simulink model "svpwm_inv_Motor_new_sent_split4_myMod1_simplified_free"  (R2023a)
settings: Solver=daessc  StartTime=0.0  StopTime=1  MaxStep=2.5e-7  RelTol=1e-3
libraries: fl_lib x17, nesl_utility x11, ee_lib x1, simulink x1
settings Model: SimulationMode=rapid-accelerator  Creator=alexey  LastModifiedBy=alexey
settings SolverCC: ZeroCrossAlgorithm=Adaptive
settings OptimizationCC: ReuseModelBlockBuffer=off
settings DebuggingCC: IgnoredZcDiagnostic=none
settings GRTTargetCC: RTWCAPISignals=on  RTWCAPIParams=on

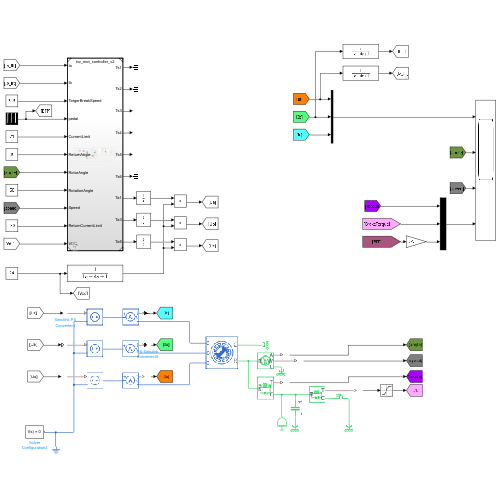
[thumbnail: Simulink's stored preview of the top-level diagram]
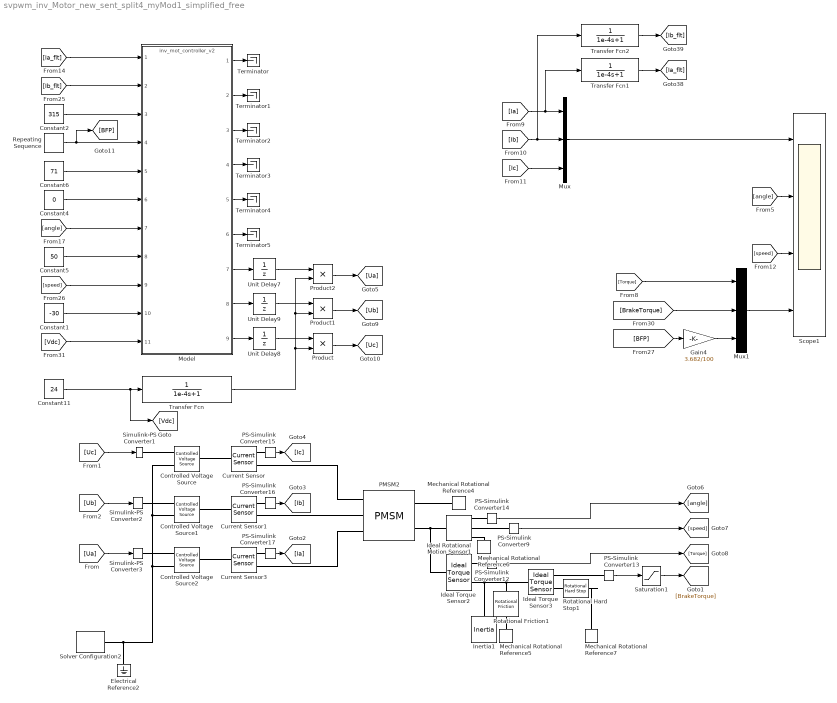
== system svpwm_inv_Motor_new_sent_split4_myMod1_simplified_free ==
  Constant1 : Constant  Value=-30
  Constant11 : Constant  Value=24
  Constant2 : Constant  Value=315
  Constant4 : Constant  Value=0
  Constant5 : Constant  Value=50
  Constant6 : Constant  Value=71
  Controlled Voltage Source : fl_lib/Electrical/Electrical Sources/Controlled Voltage Source
  Controlled Voltage Source1 : fl_lib/Electrical/Electrical Sources/Controlled Voltage Source
  Controlled Voltage Source2 : fl_lib/Electrical/Electrical Sources/Controlled Voltage Source
  Current Sensor : fl_lib/Electrical/Electrical Sensors/Current Sensor
  Current Sensor1 : fl_lib/Electrical/Electrical Sensors/Current Sensor
  Current Sensor3 : fl_lib/Electrical/Electrical Sensors/Current Sensor
  Electrical Reference2 : fl_lib/Electrical/Electrical Elements/Electrical Reference
  Gain4 : Gain  Gain=3.682/100
  Ideal Rotational Motion Sensor1 : fl_lib/Mechanical/Mechanical Sensors/Ideal Rotational Motion Sensor  reference=foundation.enum.MeasurementReference.difference  acceleration_port=false  velocity_port=true  position_port=true  wrap_angle=false  offset=0 rad
  Ideal Torque Sensor2 : fl_lib/Mechanical/Mechanical Sensors/Ideal Torque Sensor
  Ideal Torque Sensor3 : fl_lib/Mechanical/Mechanical Sensors/Ideal Torque Sensor
  Inertia1 : fl_lib/Mechanical/Rotational Elements/Inertia  inertia=3e-5 kg*m^2  num_ports=foundation.enum.numPorts2.one  w_specify=on  w_priority=High  w=0 rad/s  w_nominal_specify=off  w_nominal_unit=rad/s  w_nominal_value=1  t_specify=off  t_priority=None  t=0 N*m  t_nominal_specify=off  t_nominal_unit=N*m  t_nominal_value=1
  Mechanical Rotational Reference{4..7} (4 alike) : fl_lib/Mechanical/Rotational Elements/Mechanical Rotational Reference
  Model : ModelReference  ModelNameDialog=inv_mot_controller_v2.slx  SimulationMode=Normal  ModelReferenceVersion=1.6
  Mux : Mux  Inputs=3
  Mux1 : Mux  Inputs=3
  PMSM2 : ee_lib/Electromechanical/Permanent Magnet/PMSM  port_option=ee.enum.threePhasePort.expanded  winding_type=ee.enum.statorconnection.delta  machine_param=ee.enum.pmsm.parameterization.constant  nPolePairs=4  pmflux_param=ee.enum.pmflux.fluxlinkage  pm_flux_linkage=0.0163 Wb  torque_constant=0.074 N*m/A  back_emf_constant=0.06 V*s/rad  stator_param=ee.enum.statorparam.LdLqL0  Ld=119 uH  Lq=167 uH  idVec=[-200, 0, 200] A  iqVec=[-200, 0, 200] A  LdMatrix=0.0002 * ones(3, 3) H  LqMatrix=0.0002 * ones(3, 3) H  PmMatrix=0.1 * ones(3, 3) Wb  ktMatrix=0.18 * ones(3, 3) N*m/A  keMatrix=0.18 * ones(3, 3) V*s/rad  L0=1e-6 uH  Ls=0.0002 H  Lm=-0.00002 H  Ms=0.00002 H  Rs=0.1 Ohm  zero_sequence=ee.enum.park.zerosequence.include  axes_param=ee.enum.rotorangle.daxis  loss_param=ee.enum.ironloss.none  losses_oc=[0, 0, 0] W  losses_sc=[0, 0, 0] W  f_losses=60 Hz  Isc_losses=95 A  J=1e-8 kg*m^2  lam=0.00005 N*m*s/rad  i_d_specify=on  i_d_priority=None  i_d=0 A  i_d_nominal_specify=off  i_d_nominal_unit=A  i_d_nominal_value=1  i_q_specify=on  i_q_priority=None  i_q=0 A  i_q_nominal_specify=off  i_q_nominal_unit=A  i_q_nominal_value=1  torque_specify=on  torque_priority=None  torque=0 N*m  torque_nominal_specify=off  torque_nominal_unit=N*m  torque_nominal_value=1  angular_velocity_specify=off  angular_velocity_priority=High  angular_velocity=0 rpm  angular_velocity_nominal_specify=off  angular_velocity_nominal_unit=rpm  angular_velocity_nominal_value=1  angular_position_specify=off  angular_position_priority=High  angular_position=0 deg  angular_position_nominal_specify=off  angular_position_nominal_unit=deg  angular_position_nominal_value=1  alpha=3.93e-3 1/K  alpha_flux=-0.001 1/K  Tmeas=298.15 K  stator_thermal_mass=100 J/K  rotor_thermal_mass=200 J/K  Rm_percent_rotor=90  Rd_percent_rotor=30  temperatureA_specify=off  temperatureA_priority=High  temperatureA=25 degC  temperatureA_nominal_specify=off  temperatureA_nominal_unit=degC  temperatureA_nominal_value=1  temperatureB_specify=off  temperatureB_priority=High  temperatureB=25 degC  temperatureB_nominal_specify=off  temperatureB_nominal_unit=degC  temperatureB_nominal_value=1  temperatureC_specify=off  temperatureC_priority=High  temperatureC=25 degC  temperatureC_nominal_specify=off  temperatureC_nominal_unit=degC  temperatureC_nominal_value=1  temperatureR_specify=off  temperatureR_priority=High  temperatureR=25 degC  temperatureR_nominal_specify=off  temperatureR_nominal_unit=degC  temperatureR_nominal_value=1
      settings: InternalSimscapePortConfiguration="{\"Bottom\":[],\"Left\":[{\"id\":\"a\",\"label\":\"a\",\"type\":\"foundation.electrical.electrical\"},{\"id\":\"b\",\"label\":\"b\",\"type\":\"foundation.electrical.electrical\"},{\"id\":\"c\",\"label\":\"c\",\"type\":\"foundation.electrical.electrical\"}],\"Right\":[{\"id\":\"R\",\"label\":\"R\",\"type\":\"foundation.mechanical.rotational.rotational\"},{\"id\":\"C\",\"label\":\"C\",\"type\":\"foundation.mechanical.rotational.rotational\"}],\"Top\":[]}"
  PS-Simulink Converter{9,12..17} (7 alike) : nesl_utility/PS-Simulink Converter  PhysicalDomain=network_engine_domain  SubClassName=ps_output  LeftPortType=input  RightPortType=output  PseudoPeriodic=off  Frequencies=[]  VectorFormat=inherit  Unit=inherit  AffineConversion=off
  Product : Product
  Product1 : Product
  Product2 : Product
  Repeating Sequence : simulink/Sources/Repeating Sequence  rep_seq_t=[0 0.4 0.6 0.61 1 1.4 1.6 1.61 2 2.05 2.08 2.081 2.5 2.501 2.8 2.9 3]  rep_seq_y="[0 100 100 0 0  15 15 0 0 55 95 0 0 100 100 70 0]"
  Rotational Friction1 : fl_lib/Mechanical/Rotational Elements/Rotational Friction  brkwy_trq=0.31 N*m  brkwy_vel=0.01 rad/s  Col_trq=0.3 N*m  visc_coef=0.001 N*m*s/rad  w_specify=off  w_priority=None  w=0 rad/s  w_nominal_specify=off  w_nominal_unit=rad/s  w_nominal_value=1  t_specify=off  t_priority=None  t=0 N*m  t_nominal_specify=off  t_nominal_unit=N*m  t_nominal_value=1
  Rotational Hard Stop1 : fl_lib/Mechanical/Rotational Elements/Rotational Hard Stop  upper_bnd=14.8*pi/7.4+0.2 rad  lower_bnd=(-2*pi) rad  model=simscape.enum.hardstop.fulldamped  stiff_up=1e6 N*m/rad  stiff_low=1e6 N*m/rad  D_up=1500 N*m*s/rad  D_low=1500 N*m*s/rad  transition=0.001 rad  coeff_rest=0.7  w_tol=0.1 rad/s  trq_tol=0.001 N*m  phi_specify=off  phi_priority=High  phi=0 rad  phi_nominal_specify=off  phi_nominal_unit=rad  phi_nominal_value=1  w_specify=off  w_priority=None  w=0 rad/s  w_nominal_specify=off  w_nominal_unit=rad/s  w_nominal_value=1  t_specify=off  t_priority=None  t=0 N*m  t_nominal_specify=off  t_nominal_unit=N*m  t_nominal_value=1  M_specify=off  M_priority=None  M=0
  Saturation1 : Saturate  UpperLimit=5  LowerLimit=0
  Scope1 : Scope  NumInputPorts=4
  Simulink-PS Converter1 : nesl_utility/Simulink-PS Converter  PhysicalDomain=network_engine_domain  SubClassName=ps_input  LeftPortType=input  RightPortType=output  PseudoPeriodic=off  Frequencies=[]  NoiseDistribution=none  NoiseParameters=[]  Unit=1  AffineConversion=off  FilteringAndDerivatives=provide  SimscapeFilterOrder=1  InputFilterTimeConstant=0.001  UdotUserProvided=0
  Simulink-PS Converter2 : nesl_utility/Simulink-PS Converter  PhysicalDomain=network_engine_domain  SubClassName=ps_input  LeftPortType=input  RightPortType=output  PseudoPeriodic=off  Frequencies=[]  NoiseDistribution=none  NoiseParameters=[]  Unit=1  AffineConversion=off  FilteringAndDerivatives=provide  SimscapeFilterOrder=1  InputFilterTimeConstant=0.001  UdotUserProvided=0
  Simulink-PS Converter3 : nesl_utility/Simulink-PS Converter  PhysicalDomain=network_engine_domain  SubClassName=ps_input  LeftPortType=input  RightPortType=output  PseudoPeriodic=off  Frequencies=[]  NoiseDistribution=none  NoiseParameters=[]  Unit=1  AffineConversion=off  FilteringAndDerivatives=provide  SimscapeFilterOrder=1  InputFilterTimeConstant=0.001  UdotUserProvided=0
  Solver Configuration2 : nesl_utility/Solver Configuration  PhysicalDomain=network_engine_domain  SubClassName=solver  LeftPortType=input  RightPortType=generic  Tones=[]  Harmonics=[]  SimulateNoise=off  Profile=off  UseLocalSampling=off  EnableSwitchedLinearOptims=on  FrequencyDomain=off  UseCCode=off  RelTol=0.001  AbsTol=0.001  MinStep=1e-09  ToWorkspace=off  RevertToSquareIcSolve=off  NumHomotopyIterations=100  PhasorMode=off  PhasorModeNumHarmonics=1  ConsistencySolver=NEWTON_XTOL_AFTER_FTOL  IndexReductionMethod=DerivativeReplacement  DoDC=off  ResidualTolerance=1e-09  ConsistencyTolSource=GLOBAL  ConsistencyAbsTol=0.001  ConsistencyRelTol=0.001  ConsistencyTolFactor=0.001  UseLocalSolver=off  LocalSolverChoice=NE_BACKWARD_EULER_ADVANCER  ResolveIndetEquations=on  FunctionEvalNumThread=1  LocalSolverSampleTime=0.001  DoFixedCost=off  MaxNonlinIter=3  MaxModeIter=2  ComputeImpulses=off  ImpulseIterations=2  LinearAlgebra=auto  LinearAlgebraNumThread=0  EquationFormulation=NE_TIME_EF  DelaysMemoryBudget=1024  AutomaticFiltering=on  FilteringTimeConstant=0.001  PartitionStorageMethod=AS_NEEDED  PartitionMemoryBudget=1024  PartitionMethod=ROBUST
  Terminator{,1..5} (6 alike) : Terminator
  Transfer Fcn : TransferFcn  Denominator=[1e-4 1]
  Transfer Fcn1 : TransferFcn  Denominator=[1e-4 1]
  Transfer Fcn2 : TransferFcn  Denominator=[1e-4 1]
  Unit Delay7 : UnitDelay  SampleTime=1e-6  HasFrameUpgradeWarning=on
  Unit Delay8 : UnitDelay  SampleTime=1e-6  HasFrameUpgradeWarning=on
  Unit Delay9 : UnitDelay  SampleTime=1e-6  HasFrameUpgradeWarning=on
  wires:
  [Torque] -> Mux1/1
  [Ia] -> Transfer Fcn1/1, Mux/1
  [Ib] -> Transfer Fcn2/1, Mux/2
  [Ic] -> Mux/3
  [angle] -> Scope1/2
  [speed] -> Scope1/3
  Mux1/1 -> Scope1/4
  Gain4/1 -> Mux1/3
  [BrakeTorque] -> Mux1/2
  Model/1 -> Terminator/1
  Mux/1 -> Scope1/1
  Transfer Fcn1/1 -> [Ia_flt]
  Transfer Fcn2/1 -> [Ib_flt]
  [Ia_flt] -> Model/1
  [Ib_flt] -> Model/2
  Constant2/1 -> Model/3
  Repeating Sequence/1 -> [BFP], Model/4
  Constant6/1 -> Model/5
  Constant4/1 -> Model/6
  [angle] -> Model/7
  Constant5/1 -> Model/8
  [speed] -> Model/9
  Constant1/1 -> Model/10
  [Vdc] -> Model/11
  Model/2 -> Terminator1/1
  Model/3 -> Terminator2/1
  Model/4 -> Terminator3/1
  Model/5 -> Terminator4/1
  Model/6 -> Terminator5/1
  Saturation1/1 -> [BrakeTorque]
  PS-Simulink Converter13/1 -> Saturation1/1
  PS-Simulink Converter12/1 -> [Torque]
  PS-Simulink Converter9/1 -> [speed]
  PS-Simulink Converter14/1 -> [angle]
  Model/9 -> Unit Delay8/1
  Model/8 -> Unit Delay9/1
  Model/7 -> Unit Delay7/1
  PS-Simulink Converter15/1 -> [Ic]
  PS-Simulink Converter16/1 -> [Ib]
  PS-Simulink Converter17/1 -> [Ia]
  Unit Delay7/1 -> Product2/1
  Unit Delay8/1 -> Product/1
  Unit Delay9/1 -> Product1/1
  Transfer Fcn/1 -> Product2/2, Product1/2, Product/2
  Constant11/1 -> [Vdc], Transfer Fcn/1
  Product2/1 -> [Ua]
  Product1/1 -> [Ub]
  Product/1 -> [Uc]
  [Ua] -> Simulink-PS Converter3/1
  [Ub] -> Simulink-PS Converter2/1
  [Uc] -> Simulink-PS Converter1/1
  [BFP] -> Gain4/1
  connections:
  Controlled Voltage Source1/RConn2 -- Solver Configuration2/RConn1 -- Electrical Reference2/LConn1 -- Controlled Voltage Source2/RConn2 -- Controlled Voltage Source/RConn2
  Ideal Torque Sensor2/LConn1 -- Ideal Rotational Motion Sensor1/LConn1 -- PMSM2/RConn1
  Rotational Friction1/LConn1 -- Inertia1/LConn1 -- Ideal Torque Sensor2/RConn1 -- Ideal Torque Sensor3/LConn1
  Mechanical Rotational Reference4/LConn1 -- PMSM2/RConn2
  Ideal Rotational Motion Sensor1/RConn1 -- Mechanical Rotational Reference6/LConn1
  Rotational Friction1/RConn1 -- Mechanical Rotational Reference5/LConn1
  Ideal Rotational Motion Sensor1/RConn3 -- PS-Simulink Converter14/LConn1
  PS-Simulink Converter9/LConn1 -- Ideal Rotational Motion Sensor1/RConn2
  Rotational Hard Stop1/RConn1 -- Mechanical Rotational Reference7/LConn1
  PS-Simulink Converter12/LConn1 -- Ideal Torque Sensor2/RConn2
  Ideal Torque Sensor3/RConn1 -- Rotational Hard Stop1/LConn1
  Ideal Torque Sensor3/RConn2 -- PS-Simulink Converter13/LConn1
  Current Sensor3/RConn2 -- PMSM2/LConn1
  Current Sensor1/RConn2 -- PMSM2/LConn2
  Current Sensor/RConn2 -- PMSM2/LConn3
  Simulink-PS Converter1/RConn1 -- Controlled Voltage Source/RConn1
  Simulink-PS Converter2/RConn1 -- Controlled Voltage Source1/RConn1
  Simulink-PS Converter3/RConn1 -- Controlled Voltage Source2/RConn1
  Controlled Voltage Source/LConn1 -- Current Sensor/LConn1
  PS-Simulink Converter17/LConn1 -- Current Sensor3/RConn1
  Current Sensor1/RConn1 -- PS-Simulink Converter16/LConn1
  Current Sensor/RConn1 -- PS-Simulink Converter15/LConn1
  Current Sensor1/LConn1 -- Controlled Voltage Source1/LConn1
  Controlled Voltage Source2/LConn1 -- Current Sensor3/LConn1
